simulink model "class_5_2D"  (R2023b)
settings: Solver=VariableStepAuto  StartTime=0.0  StopTime=10.0  RelTol=1e-3
undefined symbols (not defined in the file): den, num, tSample
settings Model: Creator=klysm  LastModifiedBy=klysm

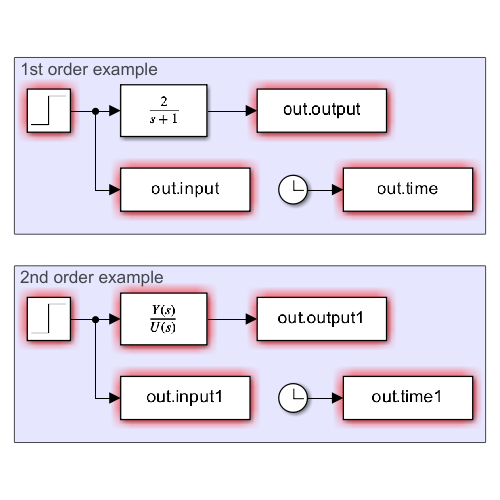
[thumbnail: Simulink's stored preview of the top-level diagram]
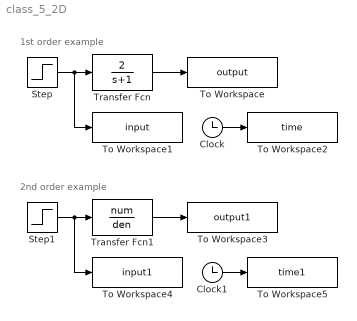
== system class_5_2D ==
  note: 2nd order example
  note: 1st order example
  Clock : Clock
  Clock1 : Clock
  Step : Step  Time=0  SampleTime=tSample
  Step1 : Step  Time=0  SampleTime=tSample
  To Workspace : ToWorkspace  VariableName=output  SampleTime=tSample
  To Workspace1 : ToWorkspace  VariableName=input  SampleTime=tSample
  To Workspace2 : ToWorkspace  VariableName=time  SampleTime=tSample
  To Workspace3 : ToWorkspace  VariableName=output1  SampleTime=tSample
  To Workspace4 : ToWorkspace  VariableName=input1  SampleTime=tSample
  To Workspace5 : ToWorkspace  VariableName=time1  SampleTime=tSample
  Transfer Fcn : TransferFcn  Numerator=2  Denominator=[1 1]
  Transfer Fcn1 : TransferFcn  Numerator=num  Denominator=den
  wires:
  Step/1 -> To Workspace1/1, Transfer Fcn/1
  Transfer Fcn/1 -> To Workspace/1
  Clock/1 -> To Workspace2/1
  Clock1/1 -> To Workspace5/1
  Transfer Fcn1/1 -> To Workspace3/1
  Step1/1 -> To Workspace4/1, Transfer Fcn1/1
